simulink model "PID"  (R2025a)
settings: Solver=FixedStepAuto  StartTime=0.0  StopTime=0.25  FixedStep=1e-3  RelTol=1e-3  AbsTol=1e-3
InitFcn:
  | init_params
undefined symbols (not defined in the file): k_d, k_i, k_p, SP
libraries: fl_lib x7, nesl_utility x3
settings Model: PacingRate=0.010000  Creator=alexpoulin  LastModifiedBy=alexpoulin
settings SolverCC: AutoScaleAbsTol=off  AlgebraicLoopSolver=TrustRegion  MaxZcPerStep=1.0
settings DebuggingCC: UnconnectedInputMsg=warning  UnconnectedOutputMsg=warning  UnconnectedLineMsg=warning  SymbolicDimsDataTypeCodeGenerationDiagnostic=none
settings ModelReferenceCC: EnableRefExpFcnMdlSchedulingChecks=on
settings SFSimCC: CustomCodeUndefinedFunction=UseInterfaceOnly
settings RTWCC: GPUComputeCapability=3.5  DLArmComputeVersion=19.05
settings SimscapeCC: SimscapeLogType=all  SimscapeLogSimulationStatistics=on  SimscapeLogToSDI=on  SimscapeLogDataHistory=10000.0

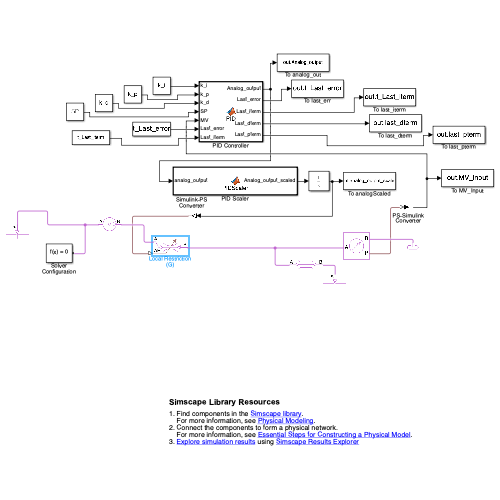
[thumbnail: Simulink's stored preview of the top-level diagram]
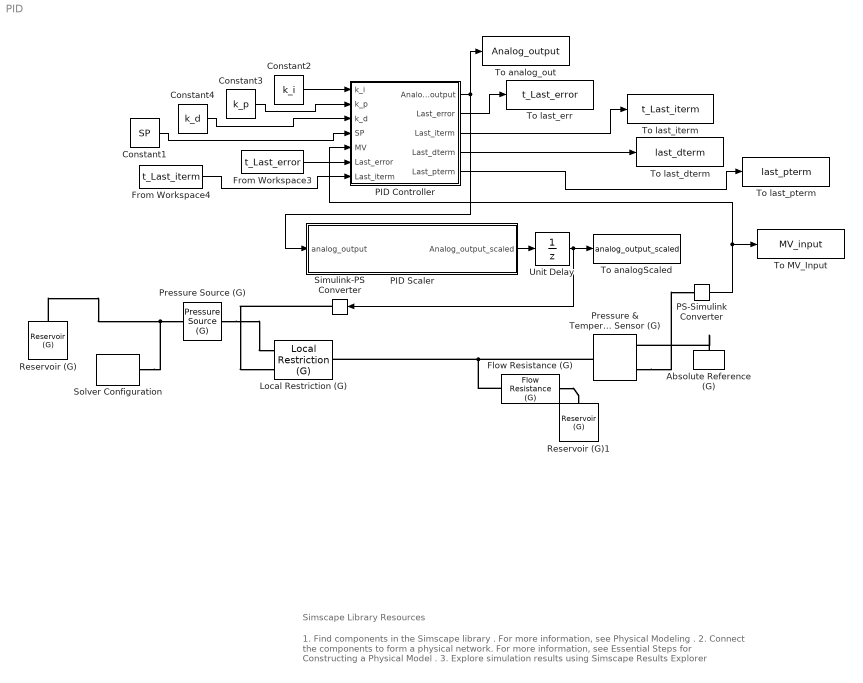
== system PID ==
  note: 1. Find components in the Simscape library .
      | For more information, see Physical Modeling .
      | 2. Connect the components to form a physical network.
      | For more information, see Essential Steps for Constructing a Physical Model .
      | 3. Explore simulation results using Simscape Results Explorer
  note: Simscape Library Resources
  Absolute Reference (G) : fl_lib/Gas/Elements/Absolute Reference (G)
      settings: InternalSimscapePortConfiguration="{\"Bottom\":[],\"Left\":[{\"id\":\"A\",\"label\":\"\",\"type\":\"foundation.gas.gas\"}],\"Right\":[],\"Top\":[]}"
  Constant1 : Constant  Value=SP
  Constant2 : Constant  Value=k_i
  Constant3 : Constant  Value=k_p
  Constant4 : Constant  Value=k_d
  Flow Resistance (G) : fl_lib/Gas/Elements/Flow Resistance (G)  delta_p_nominal=1 psi  mdot_nominal=0.1 kg/s  rho_nominal=0 kg/m^3  area=0.01 m^2  laminar_fraction=1e-3
      settings: InternalSimscapePortConfiguration="{\"Bottom\":[],\"Left\":[{\"id\":\"A\",\"label\":\"A\",\"type\":\"foundation.gas.gas\"}],\"Right\":[{\"id\":\"B\",\"label\":\"B\",\"type\":\"foundation.gas.gas\"}],\"Top\":[]}"
  From Workspace3 : FromWorkspace  VariableName=t_Last_error
  From Workspace4 : FromWorkspace  VariableName=t_Last_iterm
  Local Restriction (G) : fl_lib/Gas/Elements/Local Restriction (G)  restriction_type=foundation.enum.restriction_type.variable  restriction_area=0.0099 m^2  min_area=1e-6 m^2  max_area=0.009 m^2  area=0.01 m^2  Cd=0.64  B_lam=0.999
      settings: InternalSimscapePortConfiguration="{\"Bottom\":[],\"Left\":[{\"id\":\"A\",\"label\":\"A\",\"type\":\"foundation.gas.gas\"},{\"id\":\"area_in\",\"label\":\"AR\",\"type\":\"input\"}],\"Right\":[{\"id\":\"B\",\"label\":\"B\",\"type\":\"foundation.gas.gas\"}],\"Top\":[]}"
  PID Controller : MATLAB Function  TreatAsAtomicUnit=on
  PID Scaler : MATLAB Function  TreatAsAtomicUnit=on
  PS-Simulink Converter : nesl_utility/PS-Simulink Converter  PhysicalDomain=network_engine_domain  SubClassName=ps_output  LeftPortType=input  RightPortType=output  PseudoPeriodic=off  Frequencies=[]  VectorFormat=inherit  Unit=Pa  AffineConversion=off
  Pressure & Temperature Sensor (G) : fl_lib/Gas/Sensors/Pressure & Temperature Sensor (G)  reference=foundation.enum.MeasurementReference.difference  pressure=true  pressure_spec=foundation.enum.PressureMeasementSpec.Absolute  temperature=false
      settings: InternalSimscapePortConfiguration="{\"Bottom\":[],\"Left\":[{\"id\":\"A\",\"label\":\"A\",\"type\":\"foundation.gas.gas\"}],\"Right\":[{\"id\":\"B\",\"label\":\"B\",\"type\":\"foundation.gas.gas\"},{\"id\":\"P\",\"label\":\"P\",\"type\":\"output\"}],\"Top\":[]}"
  Pressure Source (G) : fl_lib/Gas/Sources/Pressure Source (G)  source_type=foundation.enum.constant_controlled.constant  pressure_differential=0 psi  power_spec=foundation.enum.power_spec.isentropic  area_A=0.01 m^2  area_B=0.01 m^2
      settings: InternalSimscapePortConfiguration="{\"Bottom\":[],\"Left\":[{\"id\":\"A\",\"label\":\"A\",\"type\":\"foundation.gas.gas\"}],\"Right\":[{\"id\":\"B\",\"label\":\"B\",\"type\":\"foundation.gas.gas\"}],\"Top\":[]}"
  Reservoir (G) : fl_lib/Gas/Elements/Reservoir (G)  pressure_spec=foundation.enum.pressure_spec.specified  reservoir_pressure=1000 psi  reservoir_temperature=293.15 K  area_A=0.01 m^2
  Reservoir (G)1 : fl_lib/Gas/Elements/Reservoir (G)  pressure_spec=foundation.enum.pressure_spec.atmospheric  reservoir_pressure=0.101325 MPa  reservoir_temperature=293.15 K  area_A=0.01 m^2
  Simulink-PS Converter : nesl_utility/Simulink-PS Converter  PhysicalDomain=network_engine_domain  SubClassName=ps_input  LeftPortType=input  RightPortType=output  PseudoPeriodic=off  Frequencies=[]  NoiseDistribution=none  NoiseParameters=[]  Unit=1  AffineConversion=off  FilteringAndDerivatives=provide  SimscapeFilterOrder=1  InputFilterTimeConstant=0.001  UdotUserProvided=0
  Solver Configuration : nesl_utility/Solver Configuration  PhysicalDomain=network_engine_domain  SubClassName=solver  LeftPortType=input  RightPortType=generic  Tones=[]  Harmonics=[]  SimulateNoise=off  Profile=off  UseLocalSampling=off  EnableSwitchedLinearOptims=on  FrequencyDomain=off  UseCCode=off  RelTol=0.001  AbsTol=1e-06  MinStep=1e-09  ToWorkspace=off  RevertToSquareIcSolve=off  NumHomotopyIterations=100  PhasorMode=off  PhasorModeNumHarmonics=1  ConsistencySolver=NEWTON_XTOL_AFTER_FTOL  IndexReductionMethod=DerivativeReplacement  DoDC=off  ResidualTolerance=1e-09  ConsistencyTolSource=GLOBAL  ConsistencyAbsTol=0.001  ConsistencyRelTol=0.001  ConsistencyTolFactor=0.001  UseLocalSolver=off  LocalSolverChoice=NE_BACKWARD_EULER_ADVANCER  ResolveIndetEquations=on  FunctionEvalNumThread=1  LocalSolverSampleTime=0.001  DoFixedCost=off  MaxNonlinIter=3  MaxModeIter=2  ComputeImpulses=off  ImpulseIterations=2  LinearAlgebra=auto  LinearAlgebraNumThread=0  EquationFormulation=NE_TIME_EF  DelaysMemoryBudget=1024  AutomaticFiltering=on  FilteringTimeConstant=0.001  PartitionStorageMethod=AS_NEEDED  PartitionMemoryBudget=1024  PartitionMethod=ROBUST  MultibodyUseLocalSolver=off  MultibodyLocalSolverChoice=ODE1  MultibodyLocalSolverSampleTime=0.001
  To MV_Input : ToWorkspace  VariableName=MV_input  SaveFormat=Timeseries  SampleTime=-1
  To analogScaled : ToWorkspace  VariableName=analog_output_scaled  SaveFormat=Timeseries  SampleTime=-1
  To analog_out : ToWorkspace  VariableName=Analog_output  SaveFormat=Timeseries  SampleTime=-1
  To last_dterm : ToWorkspace  VariableName=last_dterm  SaveFormat=Timeseries  SampleTime=-1
  To last_err : ToWorkspace  VariableName=t_Last_error  SaveFormat=Timeseries  SampleTime=-1
  To last_iterm : ToWorkspace  VariableName=t_Last_iterm  SaveFormat=Timeseries  SampleTime=-1
  To last_pterm : ToWorkspace  VariableName=last_pterm  SaveFormat=Timeseries  SampleTime=-1
  Unit Delay : UnitDelay  SampleTime=-1  HasFrameUpgradeWarning=on
  wires:
  PID Controller/3(Last_iterm) -> To last_iterm/1
  PID Controller/1(Analog_output) -> To analog_out/1, PID Scaler/1(analog_output)
  PID Controller/2(Last_error) -> To last_err/1
  Constant1/1 -> PID Controller/4(SP)
  Constant2/1 -> PID Controller/1(k_i)
  Constant4/1 -> PID Controller/3(k_d)
  Constant3/1 -> PID Controller/2(k_p)
  From Workspace3/1 -> PID Controller/6("Last_error ")
  From Workspace4/1 -> PID Controller/7("Last_iterm ")
  Unit Delay/1 -> To analogScaled/1, Simulink-PS Converter/1
  PID Scaler/1(Analog_output_scaled) -> Unit Delay/1
  PS-Simulink Converter/1 -> PID Controller/5(MV), To MV_Input/1
  PID Controller/5(Last_pterm) -> To last_pterm/1
  PID Controller/4(Last_dterm) -> To last_dterm/1
  connections:
  Solver Configuration/RConn1 -- Reservoir (G)/LConn1 -- Pressure Source (G)/LConn1
  Simulink-PS Converter/RConn1 -- Local Restriction (G)/LConn2
  Pressure Source (G)/RConn1 -- Local Restriction (G)/LConn1
  Pressure & Temperature Sensor (G)/LConn1 -- Flow Resistance (G)/LConn1 -- Local Restriction (G)/RConn1
  Pressure & Temperature Sensor (G)/RConn2 -- PS-Simulink Converter/LConn1
  Absolute Reference (G)/LConn1 -- Pressure & Temperature Sensor (G)/RConn1
  Flow Resistance (G)/RConn1 -- Reservoir (G)1/LConn1

== matlab function PID/PID Controller ==
  data: k_i input; k_p input; k_d input; SP input; MV input; Last_error input; Analog_output output; Last_iterm input; Last_error output; Last_iterm output; Last_dterm output; Last_pterm output
function [Analog_output, Last_error, Last_iterm, Last_dterm, Last_pterm] = PID(k_i, k_p, k_d, SP, MV, Last_error, Last_iterm)
% t function [Analog_output, Last_error, Last_iterm, Last_dterm, Last_pterm]= PID(k_i, k_p, k_d, SP, MV, Last_error, Last_iterm)

%convert MV from Pa to PSI
% MV_psi = MV * 0.0001450377;


error = SP - MV;
pterm = k_p * error;
iterm = k_i * error + Last_iterm;
dterm = k_d * (error - Last_error);
PID_output = (pterm + iterm + dterm);% * k;
Analog_output = PID_output; %should be between 1e-10 and 0.009
% Analog_output = 1;
Last_error = error;
Last_iterm = iterm;

%not used but just to see
Last_dterm = dterm;
Last_pterm = pterm;


end

== matlab function PID/PID Scaler ==
  data: analog_output input; Analog_output_scaled output
function Analog_output_scaled = PIDScaler(analog_output)

% Define limits
A_min = 1e-6;
A_max = 0.009;

% Normalize PID output
% S = max(min(analog_output, 1), 0);  % Clamp to [0, 1]

% S = 1 - S; %invert

% Scale to physical area range
% Analog_output_scaled = A_min + S * (A_max - A_min);
Analog_output_scaled = max(min(analog_output, A_max), A_min);


end
